simulink model "Feeder_IREQ_2012"  (Simulink 8.3)
settings: Solver=FixedStepDiscrete  StartTime=0.0  StopTime=100  FixedStep=50e-6  RelTol=1e-3
InitFcn:
  | Ts= 50e-6;
undefined symbols (not defined in the file): D11, Delta, DiscIntNeverNeededParam, Ion, kaimal_num, Lithium, u0
libraries: powerlib x62, powerlib_extras x49, simulink x14, simulink_extras x12, sps_avr x2, electricdrivelib x1
(part 1 of 5)
settings Model: Creator=dmasca1  LastModifiedBy=inovic  SimulationMode=accelerator
settings DataIOCC: SignalLoggingSaveFormat=Dataset  InspectSignalLogs=on
settings OptimizationCC: ExpressionDepthLimit=2147483647
settings DebuggingCC: UnconnectedInputMsg=none  UnconnectedOutputMsg=none  UnconnectedLineMsg=none  FrameProcessingCompatibilityMsg=error
settings GRTTargetCC: CombineOutputUpdateFcns=on  GRTInterface=off
settings ConfigComp: CovMetricSettings=dw  CovHtmlReporting=on  CovSaveCumulativeToWorkspaceVar=on  CovSaveSingleToWorkspaceVar=on  CovExternalEMLEnable=off

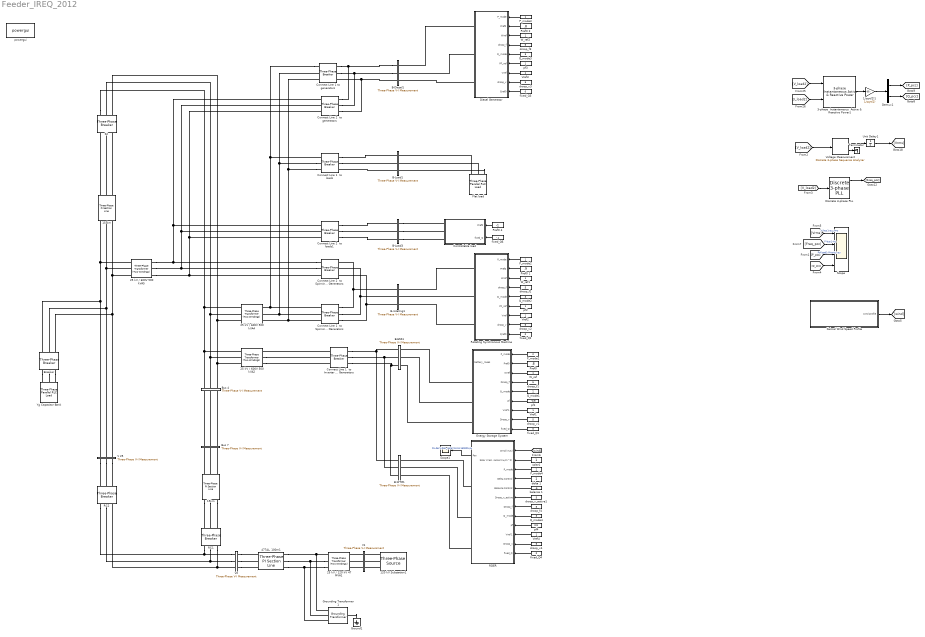
== system Feeder_IREQ_2012 ==
  " Yg Capacitor Bank" : powerlib/Elements/Three-Phase Parallel RLC Load  LConnTagsString=A|B|C  Configuration=Y (grounded)  NominalVoltage=25e3  NominalFrequency=60  ActivePower=0  InductivePower=0  CapacitivePower=5.9376e+5  Measurements=None  LoadType=constant Z
  1/sqrt(2)1 : Gain  Gain=1/sqrt(2)
  120 kV Substation1 : powerlib/Electrical Sources/Three-Phase Source  Voltage=121.2e3  PhaseAngle=0  Frequency=60  InternalConnection=Yg  SpecifyImpedance=off  Resistance=0  Inductance=0.2652582385e-3  ShortCircuitLevel=100e6  BaseVoltage=25e3  XRratio=7  BusType=swing  Pref=0  Qref=0  Qmin=-inf  Qmax=inf
  15 km : powerlib/Elements/Three-Phase PI Section Line  LConnTagsString=a|b|c  RConnTagsString=A|B|C  Frequency=60  Resistances=[ 0.12 0.29]  Inductances="[ 1.0159e-3  4.9073e-3]"  Capacitances=[1.1671e-8 3.7136e-9]  Length=15
  15km : powerlib/Elements/Three-Phase PI Section Line  LConnTagsString=a|b|c  RConnTagsString=A|B|C  Frequency=60  Resistances=[ 0.12 0.29]  Inductances="[ 1.0159e-3  4.9073e-3]"  Capacitances=[1.1671e-8 3.7136e-9]  Length=15
  25 kV / 120 kV 47 MVA1 : powerlib/Elements/Three-Phase Transformer (Two Windings)  Winding1Connection=Yg  UNITS=pu  NominalPower=[ 47e6 , 60 ]  Winding1=[ 25e3 , 0.025/30 , 0.025]  Winding2Connection=Delta (D11)  Winding2=[ 120e3 , 0.025/30 , 0.025]  SetSaturation=off  Rm=500  Lm=500  Saturation=[ 0,0; 0.002, 1; 0.01, 1.075; 0.025, 1.15; 0.05, 1.2; 0.1, 1.23; 2.0, 1.72 ]  Hysteresis=off  DataFile='hysteresis.mat'  SetInitialFlux=off  InitialFluxes=[-4.09559498760553 4.10238458550498 -0.00678959830211837]  Measurements=None  MoreParameters=off  BreakLoop=off  DataType=off  TransfoNumber=1
  25 kV / 600V 500 kVA2 : powerlib/Elements/Three-Phase Transformer (Two Windings)  Winding1Connection=Yg  UNITS=pu  NominalPower=[ 1e6 , 60 ]  Winding1=[ 25e3 , 0.001 , 0.003]  Winding2Connection=Yg  Winding2=[ .6e3 , 0.001 , 0.003]  SetSaturation=off  Rm=500  Lm=500  Saturation=[ 0,0; 0.002, 1; 0.01, 1.075; 0.025, 1.15; 0.05, 1.2; 0.1, 1.23; 2.0, 1.72 ]  Hysteresis=off  DataFile='hysteresis.mat'  SetInitialFlux=off  InitialFluxes=[-14.5645088551278 14.2446467372562 0.319846058536584]  Measurements=None  MoreParameters=off  BreakLoop=off  DataType=off  TransfoNumber=1
  25 kV / 600V 500 kVA4 : powerlib/Elements/Three-Phase Transformer (Two Windings)  Winding1Connection=Yg  UNITS=pu  NominalPower=[ 1e6 , 60 ]  Winding1=[ 25e3 , 0.001 , 0.003]  Winding2Connection=Yg  Winding2=[ .6e3 , 0.001 , 0.003]  SetSaturation=off  Rm=500  Lm=500  Saturation=[ 0,0; 0.002, 1; 0.01, 1.075; 0.025, 1.15; 0.05, 1.2; 0.1, 1.23; 2.0, 1.72 ]  Hysteresis=off  DataFile='hysteresis.mat'  SetInitialFlux=off  InitialFluxes=[-16.054288717084 15.9963868078432 0.057885949110542]  Measurements=None  MoreParameters=off  BreakLoop=off  DataType=off  TransfoNumber=1
  25 kV / 600V 500 kVA5 : powerlib/Elements/Three-Phase Transformer (Two Windings)  Winding1Connection=Yg  UNITS=pu  NominalPower=[ 1e6 , 60 ]  Winding1=[ 25e3 , 0.001 , 0.003]  Winding2Connection=Yg  Winding2=[ .6e3 , 0.001 , 0.003]  SetSaturation=off  Rm=500  Lm=500  Saturation=[ 0,0; 0.002, 1; 0.01, 1.075; 0.025, 1.15; 0.05, 1.2; 0.1, 1.23; 2.0, 1.72 ]  Hysteresis=off  DataFile='hysteresis.mat'  SetInitialFlux=off  InitialFluxes=[-16.07168869333 16.0134837471894 0.0581619685489672]  Measurements=None  MoreParameters=off  BreakLoop=off  DataType=off  TransfoNumber=1
  3-phase  Instantaneous  Active & Reactive Power1 : powerlib_extras/Measurements/3-phase  Instantaneous  Active & Reactive Power
  "477AL, 100m1" : powerlib/Elements/Three-Phase PI Section Line  LConnTagsString=a|b|c  RConnTagsString=A|B|C  Frequency=60  Resistances=[ 0.12 0.29]  Inductances="[ 1.0159e-3  4.9073e-3]"  Capacitances=[1.1671e-8 3.7136e-9]  Length=0.1
  B-Diesel1 : powerlib/Measurements/Three-Phase V-I Measurement  VoltageMeasurement=phase-to-ground  SetLabelV=on  LabelV=V_diesel  Vpu=on  VpuLL=off  CurrentMeasurement=yes  SetLabelI=on  LabelI=I_diesel  Ipu=on  Pbase=400e3  Vbase=600  OutputType=Complex  PhasorSimulation=off  PSBequivalent=0
  B-ESS1 : powerlib/Measurements/Three-Phase V-I Measurement  VoltageMeasurement=phase-to-ground  SetLabelV=on  LabelV=V_ess  Vpu=on  VpuLL=off  CurrentMeasurement=yes  SetLabelI=on  LabelI=I_ess  Ipu=on  Pbase=250e3  Vbase=600  OutputType=Complex  PhasorSimulation=off  PSBequivalent=0
  B-Load1 : powerlib/Measurements/Three-Phase V-I Measurement  VoltageMeasurement=phase-to-ground  SetLabelV=on  LabelV=V_load1  Vpu=on  VpuLL=off  CurrentMeasurement=yes  SetLabelI=on  LabelI=I_load1  Ipu=on  Pbase=3.3541e5  Vbase=600  OutputType=Complex  PhasorSimulation=off  PSBequivalent=0
  B-Load3 : powerlib/Measurements/Three-Phase V-I Measurement  VoltageMeasurement=phase-to-ground  SetLabelV=on  LabelV=V_load2  Vpu=on  VpuLL=off  CurrentMeasurement=yes  SetLabelI=on  LabelI=I_load2  Ipu=on  Pbase=350e3  Vbase=600  OutputType=Complex  PhasorSimulation=off  PSBequivalent=0
  B-WTG1 : powerlib/Measurements/Three-Phase V-I Measurement  VoltageMeasurement=phase-to-ground  SetLabelV=on  LabelV=V_wtg  Vpu=on  VpuLL=off  CurrentMeasurement=yes  SetLabelI=on  LabelI=I_wtg  Ipu=on  Pbase=250e3  Vbase=600  OutputType=Complex  PhasorSimulation=off  PSBequivalent=0
  B-rotating1 : powerlib/Measurements/Three-Phase V-I Measurement  VoltageMeasurement=phase-to-ground  SetLabelV=on  LabelV=V_rot  Vpu=on  VpuLL=off  CurrentMeasurement=yes  SetLabelI=on  LabelI=I_rot  Ipu=on  Pbase=300e3  Vbase=600  OutputType=Complex  PhasorSimulation=off  PSBequivalent=0
  Breaker : powerlib/Elements/Three-Phase Breaker  InitialState=open  SwitchA=off  SwitchB=off  SwitchC=off  SwitchTimes=[9 15]  External=off  BreakerResistance=0.001  SnubberResistance=1e9  SnubberCapacitance=inf  Measurements=None
  Bus 4 : powerlib/Measurements/Three-Phase V-I Measurement  VoltageMeasurement=phase-to-ground  SetLabelV=on  LabelV=VabcB4  Vpu=on  VpuLL=off  CurrentMeasurement=no  SetLabelI=on  LabelI=IabcB2  Ipu=on  Pbase=47e6  Vbase=25e3  OutputType=Complex  PhasorSimulation=on  PSBequivalent=0
  Bus 7 : powerlib/Measurements/Three-Phase V-I Measurement  VoltageMeasurement=phase-to-ground  SetLabelV=on  LabelV=VabcB7  Vpu=on  VpuLL=off  CurrentMeasurement=yes  SetLabelI=on  LabelI=IabcB7  Ipu=on  Pbase=47e6  Vbase=120e3  OutputType=Complex  PhasorSimulation=on  PSBequivalent=0
  Connect Line 1 to generators : powerlib/Elements/Three-Phase Breaker  InitialState=open  SwitchA=off  SwitchB=off  SwitchC=off  SwitchTimes="[4/60  10/60]"  External=off  BreakerResistance=0.001  SnubberResistance=1e6  SnubberCapacitance=inf  Measurements=None
  Connect Line 1  to Inverter Interfaced Generators : powerlib/Elements/Three-Phase Breaker  InitialState=closed  SwitchA=off  SwitchB=off  SwitchC=off  SwitchTimes="[4/60  10/60]"  External=off  BreakerResistance=0.001  SnubberResistance=1e6  SnubberCapacitance=inf  Measurements=None
  "Connect Line 1  to Spinning Generators " : powerlib/Elements/Three-Phase Breaker  InitialState=closed  SwitchA=off  SwitchB=off  SwitchC=off  SwitchTimes="[4/60  10/60]"  External=off  BreakerResistance=0.001  SnubberResistance=1e6  SnubberCapacitance=inf  Measurements=None
  Connect Line 1  to loads : powerlib/Elements/Three-Phase Breaker  InitialState=closed  SwitchA=off  SwitchB=off  SwitchC=off  SwitchTimes="[4/60  10/60]"  External=off  BreakerResistance=0.001  SnubberResistance=1e6  SnubberCapacitance=inf  Measurements=None
  Connect Line 2  to Spinning Generators : powerlib/Elements/Three-Phase Breaker  InitialState=open  SwitchA=off  SwitchB=off  SwitchC=off  SwitchTimes="[4/60  10/60]"  External=off  BreakerResistance=0.001  SnubberResistance=1e6  SnubberCapacitance=inf  Measurements=None
  Connect Line 2  to generators : powerlib/Elements/Three-Phase Breaker  InitialState=closed  SwitchA=off  SwitchB=off  SwitchC=off  SwitchTimes="[4/60  10/60]"  External=off  BreakerResistance=0.001  SnubberResistance=1e6  SnubberCapacitance=inf  Measurements=None
  Connect Line 2  to loads1 : powerlib/Elements/Three-Phase Breaker  InitialState=closed  SwitchA=off  SwitchB=off  SwitchC=off  SwitchTimes="[4/60  10/60]"  External=off  BreakerResistance=0.001  SnubberResistance=1e6  SnubberCapacitance=inf  Measurements=None
  Controllable load : Subsystem  mask{Pnom=700e3/2, Vnom=600, Pbat=575e3/2, Vbat=1100, Ebat=125e3}
      mask prompts: Pnom "Converter power [VA]"; Vnom "Nominal voltage [V]"; Pbat "Battery Power"; Vbat "Battery voltage [V]"; Ebat "Battery energy rating [kWh]"
      mask init:
      | R_RL = 0.15/50;
      | L_RL = 0.15;
      | C_var_filter = 100e3;
      | Q_filter = 100;
      | 
      | 
      | Fnom = 60;
      | Vdc = 700;
      | Mod_index_max=1.1;
      | Iq_ref_limit_time_constant=0.3; %(s)
      | Current_reg_output_limit=1.1;   %(pu)
      | Imax_grid_conv = 1.1;
      | Ts = 50e-6;
  Demux1 : Demux  Outputs=2
  Diesel Generator : Subsystem  mask{Pnom=400e3, Pmec=320e3}
      mask prompts: Pnom "Pnom [VA]"; Pmec "Pmec [W]"
  Discrete 3-phase PLL : powerlib_extras/Discrete  Control Blocks/Discrete 3-phase PLL  Fmin=0.75*60  Par_Init=[-45 60]  ParK=[60 1400 1]  Ts=Ts  AGC=off
  Energy Storage System : Subsystem  mask{Pnom=250e3, Vnom=600, Pbat=100e3, Vbat=1100, Ebat=125e3, SOC_initial=100}
      mask prompts: Pnom "Converter power [VA]"; Vnom "Nominal voltage [V]"; Pbat "Battery Power"; Vbat "Battery voltage [V]"; Ebat "Battery energy rating [kWh]"; SOC_initial "Initial State of Charge [%]"
      mask init: same as Feeder_IREQ_2012/Controllable load
  Flat load : powerlib/Elements/Three-Phase Parallel RLC Load  LConnTagsString=A|B|C  Configuration=Y (grounded)  NominalVoltage=600  NominalFrequency=60  ActivePower=300e3  InductivePower=10e3  CapacitivePower=0  Measurements=None  LoadType=constant Z
  Ground1 : powerlib/Elements/Ground  LConnTagsString=a
  Grounding Transformer 1 : powerlib/Elements/Grounding Transformer   UNITS=SI  NominalPower="[47e6   60]"  NominalVoltage=25e3  ZeroSequenceImpedance_pu=[0.025 0.75]  MagnetizationBranch_pu=[500 500]  ZeroSequenceImpedance_SI=[0.33245 9.9734]  MagnetizationBranch_SI=[6648.9 6648.9]  Measurements=None
  Kaimal Wind Speed Profile : Subsystem  mask{Mean_wind=11, Turb_int=10, D_rotor=72, roughness=340, N_nom=1800, K_gb=105, Tsample=Ts}
      mask prompts: Mean_wind "Average wind speed [m/s]"; Turb_int "Turbulence intensity [%]"; D_rotor "Rotor diameter [m]"; roughness "Length scale [m]"; N_nom "Nominal speed for generator [rpm]"; K_gb "Gearbox Ratio"; Tsample "Sample time[s]"
      mask init:
      | r = D_rotor/2;
      | random = ceil(1000.*rand(3,1));
      | trans = Turb_int/100*Mean_wind*sqrt(roughness/Mean_wind);
      | c = roughness/(2*pi*Mean_wind);
      | fs = 20;
      | [kaimal_num, kaimal_den] = bilinear([0.0182*c^2 1.3653*c 0.9846], [1.3463*c^2 3.7593*c 1], fs);
      | d = r/Mean_wind;
      | [harm0_num, harm0_den] = bilinear([4.7869*d 0.9904], [7.6823*d^2 7.3518*d 1], fs);
      | [harm3_num, harm3_den] = bilinear([0.276*d 0.0307], [0.3691*d^2 1.7722*d 1], fs);
  P_mode1 : Constant  Value=2
  P_mode2 : Constant
  P_mode3 : Constant
  P_mode4 : Constant  Value=2
  "Pref0 " : Constant  Value=.8
  Pref0 1 : Constant  Value=.9
  Pref0 2 : Constant  Value=.8
  Pref0 4 : Constant  Value=-1
  Q_mode1 : Constant  Value=2
  Q_mode2 : Constant  Value=3
  Q_mode3 : Constant  Value=3
  Q_mode4 : Constant  Value=3
  RC1 : powerlib/Elements/Three-Phase Breaker  InitialState=closed  SwitchA=off  SwitchB=off  SwitchC=off  SwitchTimes=[15]  External=off  BreakerResistance=0.001  SnubberResistance=1e6  SnubberCapacitance=inf  Measurements=None
  RC2 : powerlib/Elements/Three-Phase Breaker  InitialState=open  SwitchA=off  SwitchB=off  SwitchC=off  SwitchTimes=[600]  External=off  BreakerResistance=0.001  SnubberResistance=1e6  SnubberCapacitance=inf  Measurements=None
  RDER : Subsystem  mask{Pnom=250e3, Vnom=600, Pmec=150e3, Vdc_nom=1000}
      mask prompts: Pnom "Converter power [VA]"; Vnom "Nominal voltage [V]"; Pmec "Renewable Power [W]"; Vdc_nom "DC link voltage [V]"
      mask init:
      | R_RL = 0.15/50;
      | L_RL = 0.15;
      | C_var_filter = 100e3;
      | Q_filter = 100;
      | 
      | Kp_dc = 1.1;
      | Ki_dc = 27.5;
      | Kp_grid_side_cur_reg =1;
      | Ki_grid_side_cur_reg =50;
      | Mod_index_max=1.1;
      | Iq_ref_limit_time_constant=0.3; %(s)
      | Current_reg_output_limit=1.1;   %(pu)
      | 
      | Fnom = 60;
      | Mod_index_max=1.1;
      | Iq_ref_limit_time_constant=0.3; %(s)
      | Current_reg_output_limit=1.1;   %(pu)
      | Imax_grid_conv = 1.1;
      | Ts = 50e-6;
  Rotating Synchronous Machine : Subsystem  mask{Pnom=300e3, Pmec=150e3}
      mask prompts: Pnom "Pnom [VA]"; Pmec "Pmec [W]"
  S2 : powerlib/Elements/Three-Phase Breaker  InitialState=closed  SwitchA=off  SwitchB=off  SwitchC=off  SwitchTimes="[4/60  10/60]"  External=off  BreakerResistance=0.001  SnubberResistance=1e6  SnubberCapacitance=inf  Measurements=None
  Scope : Scope  NumInputPorts=4
  Scope1 : Scope
  Terminator : Terminator
  Unit Delay1 : UnitDelay  InitialCondition=1  SampleTime=Ts
  V 25 : powerlib/Measurements/Three-Phase V-I Measurement  VoltageMeasurement=phase-to-ground  SetLabelV=on  LabelV=V25  Vpu=on  VpuLL=off  CurrentMeasurement=no  SetLabelI=on  LabelI=IabcB2  Ipu=on  Pbase=47e6  Vbase=25e3  OutputType=Complex  PhasorSimulation=on  PSBequivalent=0
  V1 : powerlib/Measurements/Three-Phase V-I Measurement  VoltageMeasurement=phase-to-ground  SetLabelV=on  LabelV=V5  Vpu=off  VpuLL=off  CurrentMeasurement=no  SetLabelI=on  LabelI=Iabc_B1  Ipu=on  Pbase=100e6  Vbase=735e3  OutputType=Complex  PhasorSimulation=off  PSBequivalent=0
  V2 : powerlib/Measurements/Three-Phase V-I Measurement  VoltageMeasurement=phase-to-ground  SetLabelV=on  LabelV=V6  Vpu=off  VpuLL=off  CurrentMeasurement=no  SetLabelI=on  LabelI=Iabc_B1  Ipu=on  Pbase=100e6  Vbase=735e3  OutputType=Complex  PhasorSimulation=off  PSBequivalent=0
  Voltage Measurement : powerlib_extras/Discrete Measurements/Discrete 3-phase Sequence Analyzer  Freq=60  n=1  seq=Positive  Par_Init=[1 0]  Ts=50e-6
  Vref{1..4} (4 alike) : Constant
  W_ref : Constant
  W_ref1 : Constant
  W_ref2 : Constant
  balance 1 : Constant  Value=.5
  delta 1 : Constant
  droop_f{1..4} (4 alike) : Constant  Value=5
  droop_v{1..4} (4 alike) : Constant  Value=5
  droop_v_active1 : Constant  Value=5
  fixed_Q{1..4} (4 alike) : Constant  Value=0
  fixed_Q6 : Constant  Value=-.1
  pf1 : Constant  Value=-0.9
  pf2 : Constant
  pf3 : Constant
  pf4 : Constant  Value=0.9
  powergui : powerlib/powergui  Priority=1  SimulationMode=Discrete  SolverType=Tustin  SampleTime=50e-6  frequency=60  SPID=on  DisableSnubberDevices=off  DisableRonSwitches=off  DisableVfSwitches=off  SwTol=0  Interpol=off  DisplayEquations=off  Ts=10  methode=off  frequencyindice=60  Pbase=100e6  ErrMax=1e-4  Iterations=50  UnitsV=kV  UnitsW=MW  FunctionMessages=off  echomessages=off  HookPort=off  EnableUseOfTLC=off  x0status=blocks  RestoreLinks=warning  ResistiveCurrentMeasurement=off  Frange=[0:2:500]  Ylog=off  Xlog=on  ShowGrid=off  save=off  variable=ZData  structure=0  ZoomFFT=off  StartTime=0.0  cycles=1  DisplayStyle=1  fundamental=60  FreqAxis=off  MaxFrequency=1000  frequencyindicesteady=1  RmsSteady=1  display=off
  solar1 : Constant
  wires:
  Kaimal Wind Speed Profile/1(wind profile) -> [wind]
  droop_f3/1 -> Diesel Generator/4(droop_f)
  Vref3/1 -> Diesel Generator/7(Vref)
  Q_mode3/1 -> Diesel Generator/5(Q_mode)
  W_ref2/1 -> Diesel Generator/3(Wref)
  P_mode3/1 -> Diesel Generator/1(P_mode)
  pf3/1 -> Diesel Generator/6(PF_ref)
  droop_v3/1 -> Diesel Generator/8(droop_v)
  fixed_Q3/1 -> Diesel Generator/9(Qref0)
  Pref0 2/1 -> Diesel Generator/2(Pref0)
  droop_f2/1 -> Rotating Synchronous Machine/4(droop_f)
  Vref2/1 -> Rotating Synchronous Machine/7(Vref)
  Q_mode2/1 -> Rotating Synchronous Machine/5(Q_mode)
  W_ref1/1 -> Rotating Synchronous Machine/3(Wref)
  P_mode2/1 -> Rotating Synchronous Machine/1(P_mode)
  pf2/1 -> Rotating Synchronous Machine/6(PF_ref)
  droop_v2/1 -> Rotating Synchronous Machine/8(droop_v)
  fixed_Q2/1 -> Rotating Synchronous Machine/9(Qref0)
  Pref0 1/1 -> Rotating Synchronous Machine/2(Pref0)
  P_mode1/1 -> Energy Storage System/1(P_mode)
  "Pref0 "/1 -> Energy Storage System/2(Pref0)
  W_ref/1 -> Energy Storage System/3(Wref)
  Vref1/1 -> Energy Storage System/7(Vref 1)
  fixed_Q1/1 -> Energy Storage System/9(fixed_Q)
  pf1/1 -> Energy Storage System/6("pf ")
  droop_f1/1 -> Energy Storage System/4(Droop_f)
  droop_v1/1 -> Energy Storage System/8(Droop_v)
  Q_mode1/1 -> Energy Storage System/5(Q_mode)
  [wind] -> RDER/1("Wind (m/s) ")
  solar1/1 -> RDER/2(Solar irradiance (kw/m^2))
  P_mode4/1 -> RDER/3(P_mode)
  delta 1/1 -> RDER/4(Delta Control)
  balance 1/1 -> RDER/5(Balance Control)
  droop_f4/1 -> RDER/7(Droop_f)
  droop_v_active1/1 -> RDER/6(Droop_v_active)
  pf4/1 -> RDER/9("pf ")
  Vref4/1 -> RDER/10(Vref 1)
  droop_v4/1 -> RDER/11(Droop_v)
  fixed_Q4/1 -> RDER/12(fixed_Q)
  Q_mode4/1 -> RDER/8(Q_mode)
  [V_load2] -> Voltage Measurement/1
  [V_load2] -> 3-phase  Instantaneous  Active & Reactive Power1/1
  [I_load2] -> 3-phase  Instantaneous  Active & Reactive Power1/2
  3-phase  Instantaneous  Active & Reactive Power1/1 -> 1/sqrt(2)1/1
  1/sqrt(2)1/1 -> Demux1/1
  Demux1/2 -> [Q_pcc]
  Demux1/1 -> [P_pcc]
  Voltage Measurement/2 -> Terminator/1
  Voltage Measurement/1 -> Unit Delay1/1
  Unit Delay1/1 -> [Vrms]
  [V_load2] -> Discrete 3-phase PLL/1
  Discrete 3-phase PLL/1 -> [Freq_pcc]
  [Vrms] -> Scope/1  "V-bus1-pu_rms"
  [Q_pcc] -> Scope/4
  [P_pcc] -> Scope/3  "Pd-load1-Priority-pu"
  [Freq_pcc] -> Scope/2  "F-bus1-Hz"
  Pref0 4/1 -> Controllable load/1(Pref0)
  fixed_Q6/1 -> Controllable load/2(fixed_Q)
  RDER/1(Pav) -> Scope1/1  "Po-der1-Ren_Solar/Wind-150000-pu"
  connections:
  Connect Line 1 to generators/LConn1 -- Connect Line 1  to loads/LConn1 -- 25 kV / 600V 500 kVA4/RConn1 -- "Connect Line 1  to Spinning Generators "/LConn1
  Connect Line 1  to loads/LConn2 -- 25 kV / 600V 500 kVA4/RConn2 -- "Connect Line 1  to Spinning Generators "/LConn2 -- Connect Line 1 to generators/LConn2
  Connect Line 1  to loads/LConn3 -- Connect Line 1 to generators/LConn3 -- "Connect Line 1  to Spinning Generators "/LConn3 -- 25 kV / 600V 500 kVA4/RConn3
  Connect Line 2  to Spinning Generators/LConn1 -- 25 kV / 600V 500 kVA5/RConn1 -- Connect Line 2  to loads1/LConn1 -- Connect Line 2  to generators/LConn1
  Connect Line 2  to Spinning Generators/LConn2 -- 25 kV / 600V 500 kVA5/RConn2 -- Connect Line 2  to loads1/LConn2 -- Connect Line 2  to generators/LConn2
  25 kV / 600V 500 kVA5/RConn3 -- Connect Line 2  to Spinning Generators/LConn3 -- Connect Line 2  to loads1/LConn3 -- Connect Line 2  to generators/LConn3
  25 kV / 600V 500 kVA4/LConn3 -- S2/RConn3 -- 25 kV / 600V 500 kVA2/LConn3 -- Bus 4/LConn3
  25 kV / 600V 500 kVA4/LConn2 -- S2/RConn2 -- 25 kV / 600V 500 kVA2/LConn2 -- Bus 4/LConn2
  S2/RConn1 -- 25 kV / 600V 500 kVA4/LConn1 -- 25 kV / 600V 500 kVA2/LConn1 -- Bus 4/LConn1
  25 kV / 600V 500 kVA5/LConn2 -- Breaker/LConn2 -- V 25/LConn2 -- 15 km/RConn2
  25 kV / 600V 500 kVA5/LConn1 -- Breaker/LConn1 -- V 25/LConn1 -- 15 km/RConn1
  B-WTG1/LConn1 -- B-ESS1/LConn1 -- Connect Line 1  to Inverter Interfaced Generators/RConn1
  B-WTG1/LConn2 -- Connect Line 1  to Inverter Interfaced Generators/RConn2 -- B-ESS1/LConn2
  B-WTG1/LConn3 -- Connect Line 1  to Inverter Interfaced Generators/RConn3 -- B-ESS1/LConn3
  V2/RConn1 -- RC2/LConn1 -- RC1/LConn1
  V2/RConn2 -- RC2/LConn2 -- RC1/LConn2
  RC2/LConn3 -- V2/RConn3 -- RC1/LConn3
  Grounding Transformer 1/LConn1 -- "477AL, 100m1"/RConn1 -- 25 kV / 120 kV 47 MVA1/LConn1
  25 kV / 120 kV 47 MVA1/LConn2 -- "477AL, 100m1"/RConn2 -- Grounding Transformer 1/LConn2
  25 kV / 120 kV 47 MVA1/LConn3 -- "477AL, 100m1"/RConn3 -- Grounding Transformer 1/LConn3
  25 kV / 600V 500 kVA5/LConn3 -- Breaker/LConn3 -- V 25/LConn3 -- 15 km/RConn3
  B-Diesel1/LConn1 -- Connect Line 1 to generators/RConn1 -- Connect Line 2  to generators/RConn1
  B-Diesel1/LConn2 -- Connect Line 1 to generators/RConn2 -- Connect Line 2  to generators/RConn2
  Connect Line 1 to generators/RConn3 -- B-Diesel1/LConn3 -- Connect Line 2  to generators/RConn3
  "Connect Line 1  to Spinning Generators "/RConn1 -- B-rotating1/LConn1 -- Connect Line 2  to Spinning Generators/RConn1
  "Connect Line 1  to Spinning Generators "/RConn2 -- B-rotating1/LConn2 -- Connect Line 2  to Spinning Generators/RConn2
  "Connect Line 1  to Spinning Generators "/RConn3 -- B-rotating1/LConn3 -- Connect Line 2  to Spinning Generators/RConn3
  Connect Line 1  to loads/RConn1 -- B-Load1/LConn1
  Connect Line 1  to loads/RConn2 -- B-Load1/LConn2
  15 km/LConn3 -- S2/LConn3
  15 km/LConn2 -- S2/LConn2
  15 km/LConn1 -- S2/LConn1
  Breaker/RConn1 -- " Yg Capacitor Bank"/LConn1
  Breaker/RConn2 -- " Yg Capacitor Bank"/LConn2
  Breaker/RConn3 -- " Yg Capacitor Bank"/LConn3
  120 kV Substation1/RConn1 -- V1/LConn1
  120 kV Substation1/RConn2 -- V1/LConn2
  120 kV Substation1/RConn3 -- V1/LConn3
  V1/RConn1 -- 25 kV / 120 kV 47 MVA1/RConn1
  V1/RConn2 -- 25 kV / 120 kV 47 MVA1/RConn2
  V1/RConn3 -- 25 kV / 120 kV 47 MVA1/RConn3
  Ground1/LConn1 -- Grounding Transformer 1/RConn1
  V2/LConn3 -- "477AL, 100m1"/LConn3
  V2/LConn2 -- "477AL, 100m1"/LConn2
  V2/LConn1 -- "477AL, 100m1"/LConn1
  V 25/RConn1 -- RC2/RConn1
  V 25/RConn2 -- RC2/RConn2
  V 25/RConn3 -- RC2/RConn3
  B-Load1/LConn3 -- Connect Line 1  to loads/RConn3
  Connect Line 2  to loads1/RConn2 -- B-Load3/LConn2
  Connect Line 2  to loads1/RConn3 -- B-Load3/LConn3
  Connect Line 2  to loads1/RConn1 -- B-Load3/LConn1
  15km/LConn1 -- Bus 7/RConn1
  15km/LConn3 -- Bus 7/RConn3
  15km/LConn2 -- Bus 7/RConn2
  15km/RConn3 -- RC1/RConn3
  15km/RConn1 -- RC1/RConn1
  15km/RConn2 -- RC1/RConn2
  Diesel Generator/RConn1 -- B-Diesel1/RConn1
  Diesel Generator/RConn2 -- B-Diesel1/RConn2
  Diesel Generator/RConn3 -- B-Diesel1/RConn3
  Rotating Synchronous Machine/RConn2 -- B-rotating1/RConn2
  Rotating Synchronous Machine/RConn1 -- B-rotating1/RConn1
  Rotating Synchronous Machine/RConn3 -- B-rotating1/RConn3
  Energy Storage System/RConn1 -- B-ESS1/RConn1
  Energy Storage System/RConn2 -- B-ESS1/RConn2
  Energy Storage System/RConn3 -- B-ESS1/RConn3
  RDER/RConn1 -- B-WTG1/RConn1
  RDER/RConn2 -- B-WTG1/RConn2
  RDER/RConn3 -- B-WTG1/RConn3
  Bus 7/LConn2 -- Bus 4/RConn2
  Bus 7/LConn3 -- Bus 4/RConn3
  Bus 7/LConn1 -- Bus 4/RConn1
  Connect Line 1  to Inverter Interfaced Generators/LConn1 -- 25 kV / 600V 500 kVA2/RConn1
  25 kV / 600V 500 kVA2/RConn3 -- Connect Line 1  to Inverter Interfaced Generators/LConn3
  25 kV / 600V 500 kVA2/RConn2 -- Connect Line 1  to Inverter Interfaced Generators/LConn2
  B-Load3/RConn1 -- Controllable load/RConn1
  B-Load3/RConn2 -- Controllable load/RConn2
  B-Load3/RConn3 -- Controllable load/RConn3
  Flat load/LConn1 -- B-Load1/RConn1
  Flat load/LConn2 -- B-Load1/RConn2
  Flat load/LConn3 -- B-Load1/RConn3

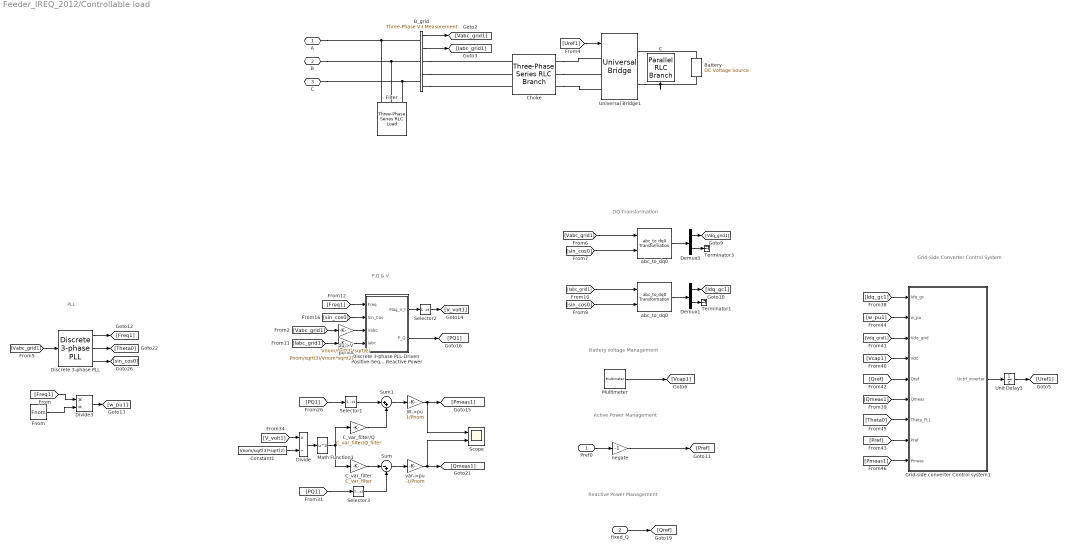
== system Feeder_IREQ_2012/Controllable load ==
  note: Battery voltage Management
  note: Grid-Side Converter
      | Control System
  note: DQ Transformation
  note: P,Q & V
  note: Reactive Power Management
  note: Active Power Management
  note: PLL
  Pref0 : Inport
  fixed_Q : Inport  Port=2
  " C " : powerlib/Elements/Parallel RLC Branch  LConnTagsString=a  RConnTagsString=__new0  BranchType=C  Resistance=1  Inductance=1e-3  SetiL0=off  InitialCurrent=0  Capacitance=3000e-6  Setx0=on  InitialVoltage=Vbat  Measurements=Branch voltage
  B_grid : powerlib/Measurements/Three-Phase V-I Measurement  VoltageMeasurement=phase-to-ground  SetLabelV=off  LabelV=Vabc  Vpu=on  VpuLL=off  CurrentMeasurement=yes  SetLabelI=off  LabelI=Iabc  Ipu=on  Pbase=Pnom  Vbase=Vnom  OutputType=Complex  PhasorSimulation=off  PSBequivalent=0
  "Battery " : powerlib/Electrical Sources/DC Voltage Source  Amplitude=Vbat  Measurements=None
  C_var_filter : Gain  Gain=C_var_filter  SaturateOnIntegerOverflow=on  OutDataTypeStr=Inherit: Same as input  ParamDataTypeStr=Inherit: Same as input
  C_var_filter/Q : Gain  Gain=C_var_filter/Q_filter  SaturateOnIntegerOverflow=on  OutDataTypeStr=Inherit: Same as input  ParamDataTypeStr=Inherit: Same as input
  "Choke " : powerlib/Elements/Three-Phase Series RLC Branch  LConnTagsString=A|B|C  RConnTagsString=A|B|C  BranchType=RL  Resistance=R_RL*Vnom^2/Pnom  Inductance=L_RL*Vnom^2/Pnom/(2*pi*Fnom)  Capacitance=[]  Measurements=None
  Constant1 : Constant  Value=Vnom/sqrt(3)*sqrt(2)
  Demux1 : Demux  Outputs=[2 1]
  Demux3 : Demux  Outputs=[2 1]
  Discrete 3-phase PLL : powerlib_extras/Discrete  Control Blocks/Discrete 3-phase PLL  Fmin=0.75*Fnom  Par_Init=[-45 Fnom]  ParK=[60 1400 1]  Ts=Ts  AGC=off
  Discrete 3-phase PLL-Driven  Positive-Sequence Active & Reactive Power : Subsystem  mask(Discrete 3-phase PLL-Driven Positive-Sequence Active & Reactive Power){Finit=Fnom, Fmin=Fnom*45/60, Par_Vinit=[Vnom/sqrt(3)*sqrt(2) 30], Par_Iinit=[Pnom/sqrt(3)/Vnom*sqrt(2) -10], Ts=Ts}
      mask prompts: Finit "Initial frequency (Hz):"; Fmin "Minimum frequency (Hz):"; Par_Vinit "Voltage initial input: [ Mag  Phase(Degrees) ]"; Par_Iinit "Current initial input: [ Mag  Phase(Degrees) ]"; Ts "Sample time:"
      mask help:
      | This discrete block measures the 3-phase active power P and reactive power Q  associated with a periodic set of 3-phase voltages and currents which may contain harmonics. P and Q are calculated by evaluating the fundamental values (positive-sequence) of the input voltages and currents with a running window over one cycle of the specified frequency (port Freq).
      |  Input port "Sin_Cos" (a two-dimension signal) provides the reference frame required for the computation.
      |
      | input 1: must give the frequency of the fundamental (Hz)
      | Input 2: must contain a  [sin(wt)  cos(wt)] two dimension signal , where w is the rotation speed (rad/s) of the reference frame used for the computation..
      | input 3: Vectorized 3-phase  instantaneous voltage (Vabc)
      | input 4: Vectorized 3-phase instantaneous current (Iabc)
      |
      | Output 1: Vector [Mag_V Mag_I] of the fundamental values (Magnitude) of the voltage & current (peak values of the positive-sequence)
      | Output 2: 3-phase PQ measurement vector [P(W) Q (var)] evaluated at the specified frequency. Current flowing into an RL circuit will produce  positive active and reactive powers.
      |
      | For the first cycle of simulation, the outputs are held constant using the values specified by the parameters "Initial input".
      | he value of the parameter "Minimum frequency" is used to determine the buffer size of the "Variable Transport Delay" block found inside this subsystem.
      mask init:
      | power_initmask();
      settings: OpenFcn=power_openblockproxy();
  Divide : Product  Inputs=*/
  Divide3 : Product  Inputs=*/
  "Filter " : powerlib/Elements/Three-Phase Series RLC Load  LConnTagsString=A|B|C  Configuration=Y (grounded)  NominalVoltage=Vnom  NominalFrequency=Fnom  ActivePower=C_var_filter/Q_filter  InductivePower=0  CapacitivePower=C_var_filter  Measurements=None  LoadType=constant Z
  Fnom : Constant  Value=Fnom
  Grid-side converter Control system1 : Subsystem
  Math Function1 : Math  Operator=square  SaturateOnIntegerOverflow=on
  Multimeter : powerlib/Measurements/Multimeter  PhasorSimulation=off  OutputType=Complex  sel=1  L=3  Gain=1  yselected={'Ub: Controllable load/ C '};  PSBOutputType=1  PSBequivalent=0  AxesSetting=[0,0.1,-100,100]  Display=0  SavedBlockNames=-11
  Scope : Scope  NumInputPorts=2
  Selector1 : Selector  InputPortWidth=2
  Selector2 : Selector  InputPortWidth=2
  Selector3 : Selector  InputPortWidth=2  Indices=2
  Sum : Sum  Inputs=|-+
  Sum1 : Sum  Inputs=|++
  Terminator1 : Terminator
  Terminator3 : Terminator
  Unit Delay3 : UnitDelay  SampleTime=Ts
  Universal Bridge1 : powerlib/Power Electronics/Universal Bridge  Arms=3  SnubberResistance=1e5  SnubberCapacitance=inf  Device=Average-model based VSC  Ron=1e-3  Lon=0  ForwardVoltages="[  0  0  ]"  ForwardVoltage=0  GTOparameters=[ 10e-6 , 20e-6 ]  IGBTparameters=[ 1e-6 , 2e-6 ]  Measurements=None  Measurements_2=None  converterType=Rectifier
  W->pu : Gain  Gain=1/Pnom  SaturateOnIntegerOverflow=on  OutDataTypeStr=Inherit: Same as input  ParamDataTypeStr=Inherit: Same as input
  abc_to_dq0 : powerlib_extras/Measurements/abc_to_dq0 Transformation
  "abc_to_dq0  " : powerlib_extras/Measurements/abc_to_dq0 Transformation
  negate : Gain  Gain=-1  SaturateOnIntegerOverflow=on  OutDataTypeStr=Inherit: Same as input  ParamDataTypeStr=Inherit: Same as input
  pu->A : Gain  Gain=Pnom/sqrt(3)/Vnom*sqrt(2)  SaturateOnIntegerOverflow=on  OutDataTypeStr=Inherit: Same as input  ParamDataTypeStr=Inherit: Same as input
  pu->V : Gain  Gain=Vnom/sqrt(3)*sqrt(2)  SaturateOnIntegerOverflow=on  OutDataTypeStr=Inherit: Same as input  ParamDataTypeStr=Inherit: Same as input
  "var->pu " : Gain  Gain=-1/Pnom  SaturateOnIntegerOverflow=on  OutDataTypeStr=Inherit: Same as input  ParamDataTypeStr=Inherit: Same as input
  A : PMIOPort  Port=1  Side=Right
  B : PMIOPort  Port=2  Side=Right
  C : PMIOPort  Port=3  Side=Right
  wires:
  Grid-side converter Control system1/1(Uctrl_inverter) -> Unit Delay3/1
  Fnom/1 -> Divide3/2
  Divide3/1 -> [w_pu1]
  [Freq1] -> Divide3/1
  Demux1/2 -> Terminator1/1
  Demux3/2 -> Terminator3/1
  "abc_to_dq0  "/1 -> Demux1/1
  abc_to_dq0/1 -> Demux3/1
  [Vabc_grid1] -> abc_to_dq0/1
  [sin_cos0] -> abc_to_dq0/2
  [sin_cos0] -> "abc_to_dq0  "/2
  B_grid/1 -> [Vabc_grid1]
  B_grid/2 -> [Iabc_grid1]
  Unit Delay3/1 -> [Uref1]
  Selector2/1 -> [V_volt1]
  Discrete 3-phase PLL-Driven  Positive-Sequence Active & Reactive Power/1(Mag_V_I) -> Selector2/1
  pu->V/1 -> Discrete 3-phase PLL-Driven  Positive-Sequence Active & Reactive Power/3(Vabc)
  [Freq1] -> Discrete 3-phase PLL-Driven  Positive-Sequence Active & Reactive Power/1(Freq)
  [sin_cos0] -> Discrete 3-phase PLL-Driven  Positive-Sequence Active & Reactive Power/2(Sin_Cos)
  pu->A/1 -> Discrete 3-phase PLL-Driven  Positive-Sequence Active & Reactive Power/4(Iabc)
  [Vabc_grid1] -> pu->V/1
  [Iabc_grid1] -> pu->A/1
  Discrete 3-phase PLL-Driven  Positive-Sequence Active & Reactive Power/2(P_Q) -> [PQ1]
  "var->pu "/1 -> Scope/2, [Qmeas1]
  [PQ1] -> Selector3/1
  W->pu/1 -> [Pmeas1], Scope/1
  [PQ1] -> Selector1/1
  [V_volt1] -> Divide/1
  Constant1/1 -> Divide/2
  Divide/1 -> Math Function1/1
  Selector3/1 -> Sum/2
  Sum/1 -> "var->pu "/1
  Math Function1/1 -> C_var_filter/Q/1, C_var_filter/1
  Selector1/1 -> Sum1/1
  Sum1/1 -> W->pu/1
  [Uref1] -> Universal Bridge1/1
  Multimeter/1 -> [Vcap1]
  [Vabc_grid1] -> Discrete 3-phase PLL/1
  Discrete 3-phase PLL/1 -> [Freq1]
  Discrete 3-phase PLL/2 -> [Theta0]
  Demux3/1 -> [Vdq_grid1]
  Demux1/1 -> [Idq_gc1]
  [Idq_gc1] -> Grid-side converter Control system1/1(Idq_gc)
  [w_pu1] -> Grid-side converter Control system1/2(w_pu)
  [Vdq_grid1] -> Grid-side converter Control system1/3(Vdq_grid)
  [Vcap1] -> Grid-side converter Control system1/4(Vdc)
  [Qref] -> Grid-side converter Control system1/5(Qref)
  [Qmeas1] -> Grid-side converter Control system1/6(Qmeas)
  [Theta0] -> Grid-side converter Control system1/7(Theta_PLL)
  [Pref] -> Grid-side converter Control system1/8(Pref)
  [Pmeas1] -> Grid-side converter Control system1/9(Pmeas)
  negate/1 -> [Pref]
  [Iabc_grid1] -> "abc_to_dq0  "/1
  fixed_Q/1 -> [Qref]
  Pref0/1 -> negate/1
  Discrete 3-phase PLL/3 -> [sin_cos0]
  C_var_filter/Q/1 -> Sum1/2
  C_var_filter/1 -> Sum/1
  connections:
  B_grid/RConn1 -- "Choke "/LConn1
  B_grid/RConn2 -- "Choke "/LConn2
  B_grid/RConn3 -- "Choke "/LConn3
  "Choke "/RConn1 -- Universal Bridge1/LConn1
  "Choke "/RConn2 -- Universal Bridge1/LConn2
  "Choke "/RConn3 -- Universal Bridge1/LConn3
  C/RConn1 -- "Filter "/LConn3 -- B_grid/LConn3
  B/RConn1 -- "Filter "/LConn2 -- B_grid/LConn2
  A/RConn1 -- "Filter "/LConn1 -- B_grid/LConn1
  Universal Bridge1/RConn2 -- "Battery "/LConn1 -- " C "/RConn1
  "Battery "/RConn1 -- Universal Bridge1/RConn1

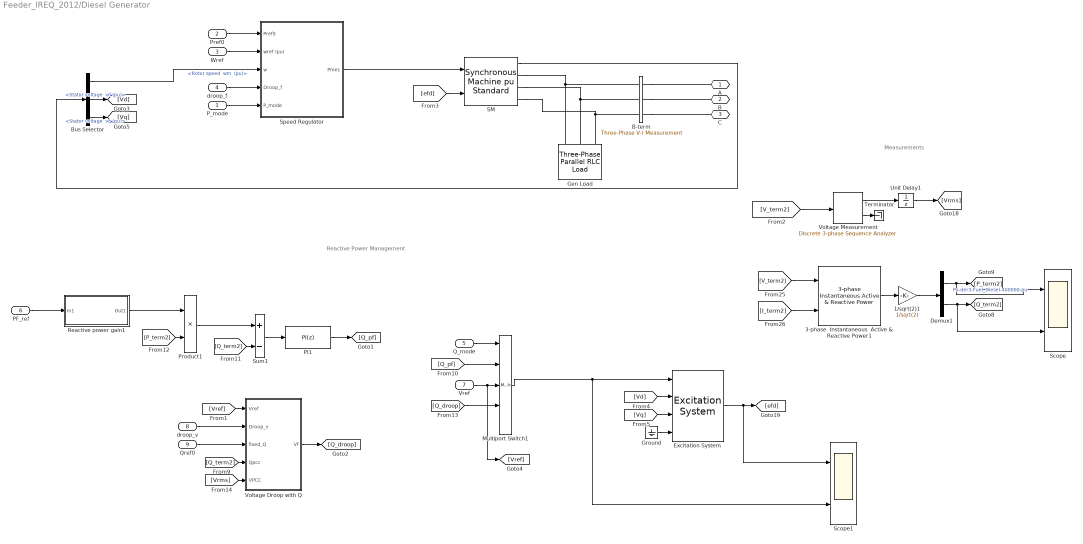
== system Feeder_IREQ_2012/Diesel Generator ==
  note: Reactive Power Management
  note: Measurements
  P_mode : Inport
  Pref0 : Inport  Port=2
  Wref : Inport  Port=3
  droop_f : Inport  Port=4
  Q_mode : Inport  Port=5
  PF_ref : Inport  Port=6
  Vref : Inport  Port=7
  droop_v : Inport  Port=8
  Qref0 : Inport  Port=9
  1/sqrt(2)1 : Gain  Gain=1/sqrt(2)
  3-phase  Instantaneous  Active & Reactive Power1 : powerlib_extras/Measurements/3-phase  Instantaneous  Active & Reactive Power
  B-term : powerlib/Measurements/Three-Phase V-I Measurement  VoltageMeasurement=phase-to-ground  SetLabelV=on  LabelV=V_term2  Vpu=on  VpuLL=off  CurrentMeasurement=yes  SetLabelI=on  LabelI=I_term2  Ipu=on  Pbase=Pnom  Vbase=600  OutputType=Complex  PhasorSimulation=off  PSBequivalent=0
  Bus Selector : BusSelector  OutputSignals="Mechanical.Rotor speed  wm  (pu),dq0 components.Stator voltage  vd (pu),dq0 components.Stator voltage  vq (pu)"
  Demux1 : Demux  Outputs=2
  "Excitation System " : sps_avr/Excitation System  tr=20e-3  reg=[ 300, 0.001 ]  exc=[ 1, 0 ]  tgr=[ 0, 0 ]  damp=[ 0.001, 0.1 ]  sat=[ 0, 0 ]  lim=[ -11.5, 11.5, 0 ]  v0="[1.0  1.28]"
  Gen Load : powerlib/Elements/Three-Phase Parallel RLC Load  LConnTagsString=A|B|C  Configuration=Y (grounded)  NominalVoltage=600  NominalFrequency=60  ActivePower=5e3  InductivePower=0  CapacitivePower=0  Measurements=None  LoadType=constant Z
  Ground : Ground
  Multiport Switch1 : MultiPortSwitch  Inputs=4  SaturateOnIntegerOverflow=on  InputSameDT=on
  PI1 : simulink/Continuous/PID Controller  Controller=PI  TimeDomain=Discrete-time  SampleTime=-1  IntegratorMethod=Forward Euler  FilterMethod=Forward Euler  Form=Parallel  P=1  I=20  D=-14.7932376623781  N=587.187356380874  InitialConditionSource=internal  InitialConditionForIntegrator=0  InitialConditionForFilter=0  ExternalReset=none  LimitOutput=on  UpperSaturationLimit=1.05  LowerSaturationLimit=.95  LinearizeAsGain=off  AntiWindupMode=back-calculation  Kb=1  TrackingMode=off  Kt=1  PParamMin=[]  PParamMax=[]  IParamMin=[]  IParamMax=[]  DParamMin=[]  DParamMax=[]  NParamMin=[]  NParamMax=[]  KbParamMin=[]  KbParamMax=[]  KtParamMin=[]  KtParamMax=[]  POutMin=[]  POutMax=[]  IOutMin=[]  IOutMax=[]  DOutMin=[]  DOutMax=[]  NOutMin=[]  NOutMax=[]  KbOutMin=[]  KbOutMax=[]  KtOutMin=[]  KtOutMax=[]  IntegratorOutMin=[]  IntegratorOutMax=[]  FilterOutMin=[]  FilterOutMax=[]  SumOutMin=[]  SumOutMax=[]  SumI1OutMin=[]  SumI1OutMax=[]  SumI2OutMin=[]  SumI2OutMax=[]  SumI3OutMin=[]  SumI3OutMax=[]  SumDOutMin=[]  SumDOutMax=[]  SaturationOutMin=[]  SaturationOutMax=[]  IntegratorContinuousStateAttributes=''  IntegratorStateMustResolveToSignalObject=off  IntegratorRTWStateStorageClass=Auto  FilterContinuousStateAttributes=''  FilterStateMustResolveToSignalObject=off  FilterRTWStateStorageClass=Auto
  Product1 : Product  RndMeth=Zero
  Reactive power gain1 : Subsystem
  SM : powerlib/Machines/Synchronous Machine pu Standard  PresetModel=No  MechanicalLoad=Mechanical power Pm  ShowDetailedParameters=on  RotorType=Round  Units=per unit standard parameters  MeasurementBus=off  NominalParameters="[ Pnom  600   60]"  Reactances1=[ 1.81, 0.3, 0.23, 1.76, 0.65, 0.25, 0.15 ]  Reactances2="[ 1.305, 0.296, 0.252, 0.474,  0.243,  0.18 ]"  dAxisTimeConstants=Open-circuit  qAxisTimeConstants=Short-circuit  TimeConstants1="[ 4.4849  0.0681  0.1  ]"  TimeConstants2=[ 8.0, 0.03, 1.0, 0.07 ]  TimeConstants3=[ 3, 0.05, 0.05 ]  TimeConstants4=[ 8.0, 0.03, 0.3371, 0.0295 ]  TimeConstants5=[ 1.01, 0.053, 0.1 ]  TimeConstants6=[ 1.3201, 0.023, 1.0, 0.07 ]  TimeConstants7=[0.012 0.003 0.003]  TimeConstants8=[ 1.3201, 0.0231, 0.3371, 0.0295 ]  StatorResistance=0.003  Mechanical=[ 1.2 0 4 ]  PolePairs=4  InitialConditions="[ 0  0  0  0  0  0  0  0  1 ]"  SetSaturation=off  Saturation=[0.6404,0.7127,0.8441,0.9214,0.9956,1.082,1.19,1.316,1.457;0.7,0.7698,0.8872,0.9466,0.9969,1.046,1.1,1.151,1.201]  LoadFlowParameters=[1,0,0,0,0]  TsPowergui=0  TsBlock=-1  IterativeModel=Trapezoidal non iterative  BusType=PV  Pref=0  Qref=0  Qmin=-inf  Qmax=inf  PLF=0  QLF=0
  Scope : Scope  NumInputPorts=2
      settings: YMin=-5~-5  YMax=5~5
  Scope1 : Scope  NumInputPorts=2
  Speed Regulator : Subsystem  mask(Diesel Engine & Governor){Tr=[0.01 0.02 0.05], Ta=[0.25 0.009 0.0384], Tlim=[0.0  1], Td=0.024, Pm0=0.25, K=40, Ts=Ts}
      mask prompts: Tr "Regulator time constants [T1 T2 ] (s) :"; Ta "Actuator time constants [T3 T4 T5] (s) :"; Tlim "Torque limits [Tmin Tmax] (pu) :"; Td "Engine time delay Td (s) :"; Pm0 "Initial value of mechanical power  Pm0 (pu) :"; K "Regulator gain K:"; Ts "Sample time"
      mask help:
      | Diesel engine and governor system. The input 1 is the measured speed, in rad/s. The input 2 is the reference speed, in pu. The output is the mechanical power.
      |
      | Controller transfer function:
      | Hc=K.(1+T1.s)/(1+T2.s)
      |
      | Throttle actuator transfer function :
      | Ha= (1+T3.s) / [ (s (1+T4.s)(1+T5.s) ]
      |
      | Motor :
      | Time delay Td
      | Inertia and viscous friction are modeled in the Synchronous generator.
      |
      | The base power used to specify the initial mechanical power (Pm0 in pu) is the nominal power of the driven generator
  Sum1 : Sum  Inputs=+-  SaturateOnIntegerOverflow=on  InputSameDT=on  OutDataTypeStr=Inherit: Same as first input
  Terminator : Terminator
  Unit Delay1 : UnitDelay  InitialCondition=1  SampleTime=Ts
  Voltage Measurement : powerlib_extras/Discrete Measurements/Discrete 3-phase Sequence Analyzer  Freq=60  n=1  seq=Positive  Par_Init=[1 0]  Ts=50e-6
  Voltage Droop with Q : Subsystem
  A : PMIOPort  Port=1  Side=Right
  B : PMIOPort  Port=2  Side=Right
  C : PMIOPort  Port=3  Side=Right
  wires:
  Qref0/1 -> Voltage Droop with Q/3(fixed_Q)
  Voltage Droop with Q/1(Vf) -> [Q_droop]
  [Q_term2] -> Voltage Droop with Q/4(Qpcc)
  Q_mode/1 -> Multiport Switch1/1
  [P_term2] -> Product1/2
  Bus Selector/1 -> Speed Regulator/3(w)  "<Rotor speed  wm  (pu)>"
  Pref0/1 -> Speed Regulator/1(Pref0)
  SM/1 -> Bus Selector/1
  [Vrms] -> Voltage Droop with Q/5(VPCC)
  [Q_droop] -> Multiport Switch1/4
  [Q_pf] -> Multiport Switch1/2
  Vref/1 -> [Vref], Multiport Switch1/3
  PI1/1 -> [Q_pf]
  Reactive power gain1/1(Out1) -> Product1/1
  droop_v/1 -> Voltage Droop with Q/2(Droop_v)
  Sum1/1 -> PI1/1
  [Q_term2] -> Sum1/2
  [efd] -> SM/2
  Product1/1 -> Sum1/1
  PF_ref/1 -> Reactive power gain1/1(In1)
  Wref/1 -> Speed Regulator/2(wref (pu))
  droop_f/1 -> Speed Regulator/4(Droop_f)
  [Vref] -> Voltage Droop with Q/1(Vref)
  P_mode/1 -> Speed Regulator/5(P_mode)
  Voltage Measurement/2 -> Terminator/1
  Voltage Measurement/1 -> Unit Delay1/1
  Unit Delay1/1 -> [Vrms]
  [V_term2] -> Voltage Measurement/1
  [V_term2] -> 3-phase  Instantaneous  Active & Reactive Power1/1
  [I_term2] -> 3-phase  Instantaneous  Active & Reactive Power1/2
  3-phase  Instantaneous  Active & Reactive Power1/1 -> 1/sqrt(2)1/1
  1/sqrt(2)1/1 -> Demux1/1
  Demux1/2 -> Scope/2, [Q_term2]
  Demux1/1 -> Scope/1, [P_term2]  "Po-der3-Fuel_Diesel-400000-pu"
  "Excitation System "/1 -> Scope1/1, [efd]
  Multiport Switch1/1 -> Scope1/2, "Excitation System "/1
  Speed Regulator/1(Pmec) -> SM/1
  Bus Selector/2 -> [Vd]  "<Stator voltage  vd (pu)>"
  Bus Selector/3 -> [Vq]  "<Stator voltage  vq (pu)>"
  [Vq] -> "Excitation System "/3
  [Vd] -> "Excitation System "/2
  Ground/1 -> "Excitation System "/4
  connections:
  B-term/LConn3 -- Gen Load/LConn3 -- SM/RConn3
  Gen Load/LConn2 -- B-term/LConn2 -- SM/RConn2
  Gen Load/LConn1 -- B-term/LConn1 -- SM/RConn1
  B-term/RConn1 -- A/RConn1
  B-term/RConn2 -- B/RConn1
  B-term/RConn3 -- C/RConn1
